simulink model "modelo_windkessel"  (R2021a)
settings: Solver=FixedStepAuto  StartTime=0.0  StopTime=20  FixedStep=0.005  RelTol=1e-3
libraries: simulink x3
settings Model: Creator=Bremdows  LastModifiedBy=Bremdows

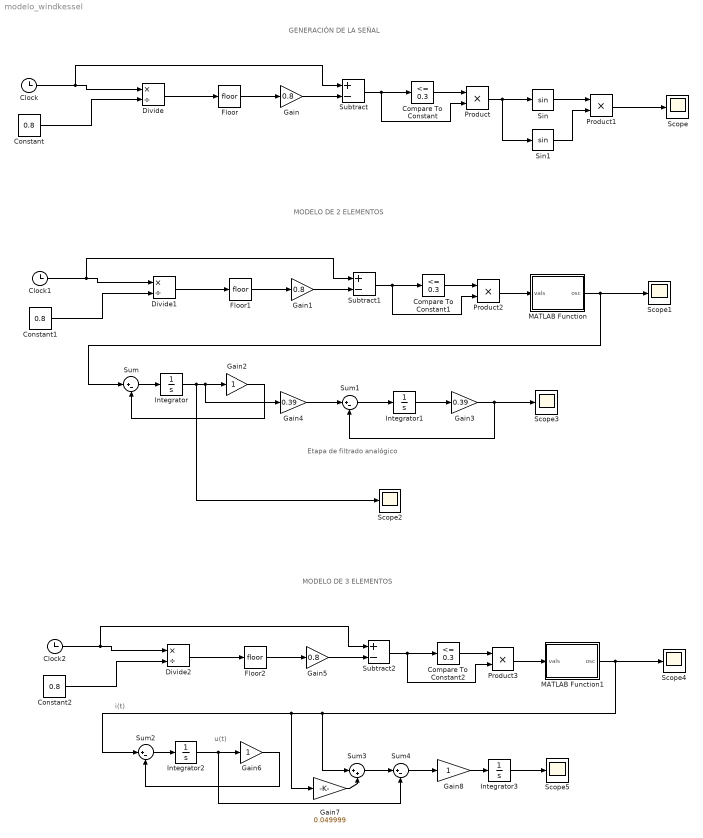
== system modelo_windkessel ==
  note: u(t)
  note: Etapa de filtrado analógico
  note: GENERACIÓN DE LA SEÑAL
  note: MODELO DE 2 ELEMENTOS
  note: MODELO DE 3 ELEMENTOS
  note: i(t)
  Clock : Clock
  Clock1 : Clock
  Clock2 : Clock
  Compare To Constant : simulink/Logic and Bit Operations/Compare To Constant  relop=<=  const=0.3  OutDataTypeStr=boolean
  Compare To Constant1 : simulink/Logic and Bit Operations/Compare To Constant  relop=<=  const=0.3  OutDataTypeStr=boolean
  Compare To Constant2 : simulink/Logic and Bit Operations/Compare To Constant  relop=<=  const=0.3  OutDataTypeStr=boolean
  Constant : Constant  Value=0.8
  Constant1 : Constant  Value=0.8
  Constant2 : Constant  Value=0.8
  Divide : Product  Inputs=*/
  Divide1 : Product  Inputs=*/
  Divide2 : Product  Inputs=*/
  Floor : Rounding
  Floor1 : Rounding
  Floor2 : Rounding
  Gain : Gain  Gain=0.8
  Gain1 : Gain  Gain=0.8
  Gain2 : Gain
  Gain3 : Gain  Gain=0.39
  Gain4 : Gain  Gain=0.39
  Gain5 : Gain  Gain=0.8
  Gain6 : Gain
  Gain7 : Gain  Gain=0.049999
  Gain8 : Gain
  Integrator : Integrator  InitialCondition=70
  Integrator1 : Integrator  InitialCondition=70
  Integrator2 : Integrator
  Integrator3 : Integrator
  MATLAB Function : MATLAB Function  TreatAsAtomicUnit=on
  MATLAB Function1 : MATLAB Function  TreatAsAtomicUnit=on
  Product{,1..3} (4 alike) : Product
  Scope{,1..5} (6 alike) : Scope
  Sin : Trigonometry
  Sin1 : Trigonometry
  Subtract : Sum  Inputs=+-
  Subtract1 : Sum  Inputs=+-
  Subtract2 : Sum  Inputs=+-
  Sum{,1..2,4} (4 alike) : Sum  Inputs=|+-
  Sum3 : Sum  Inputs=|++
  wires:
  Clock/1 -> Subtract/1, Divide/1
  Constant/1 -> Divide/2
  Divide/1 -> Floor/1
  Floor/1 -> Gain/1
  Gain/1 -> Subtract/2
  Subtract/1 -> Product/2, Compare To Constant/1
  Compare To Constant/1 -> Product/1
  Product/1 -> Sin1/1, Sin/1
  Sin/1 -> Product1/1
  Sin1/1 -> Product1/2
  Product1/1 -> Scope/1
  Constant1/1 -> Divide1/2
  Divide1/1 -> Floor1/1
  Subtract1/1 -> Product2/2, Compare To Constant1/1
  Clock1/1 -> Subtract1/1, Divide1/1
  Compare To Constant1/1 -> Product2/1
  Gain1/1 -> Subtract1/2
  Floor1/1 -> Gain1/1
  Product2/1 -> MATLAB Function/1(vals)
  MATLAB Function/1(osc) -> Scope1/1, Sum/1
  Sum/1 -> Integrator/1
  Integrator/1 -> Scope2/1, Gain4/1, Gain2/1
  Gain2/1 -> Sum/2
  Sum1/1 -> Integrator1/1
  Gain4/1 -> Sum1/1
  Integrator1/1 -> Gain3/1
  Gain3/1 -> Scope3/1, Sum1/2
  Clock2/1 -> Subtract2/1, Divide2/1
  Gain6/1 -> Sum2/2
  Product3/1 -> MATLAB Function1/1(vals)
  Floor2/1 -> Gain5/1
  Sum2/1 -> Integrator2/1
  Subtract2/1 -> Product3/2, Compare To Constant2/1
  Gain5/1 -> Subtract2/2
  Compare To Constant2/1 -> Product3/1
  Integrator2/1 -> Sum4/2, Gain6/1
  Constant2/1 -> Divide2/2
  Divide2/1 -> Floor2/1
  MATLAB Function1/1(osc) -> Scope4/1, Sum3/1, Gain7/1, Sum2/1
  Integrator3/1 -> Scope5/1
  Sum4/1 -> Gain8/1
  Gain8/1 -> Integrator3/1
  Sum3/1 -> Sum4/1
  Gain7/1 -> Sum3/2

== matlab function modelo_windkessel/MATLAB Function ==
  data: vals input; osc output
function osc = fcn(vals)
Ts = 0.3;
osc = 500*sin(pi*vals/Ts)^2;

== matlab function modelo_windkessel/MATLAB Function1 ==
  data: vals input; osc output
function osc = fcn(vals)
Ts = 0.3;
osc = 500*sin(pi*vals/Ts)^2;
